simulink model "untitled"  (R2023b)
settings: Solver=VariableStepAuto  StartTime=0.0  StopTime=500  RelTol=1e-9
values from neighbouring files (symbols this model uses):
  w0 = [w0; sol]    [vetroturbina.m]
settings Model: Creator=Anja  LastModifiedBy=Anja

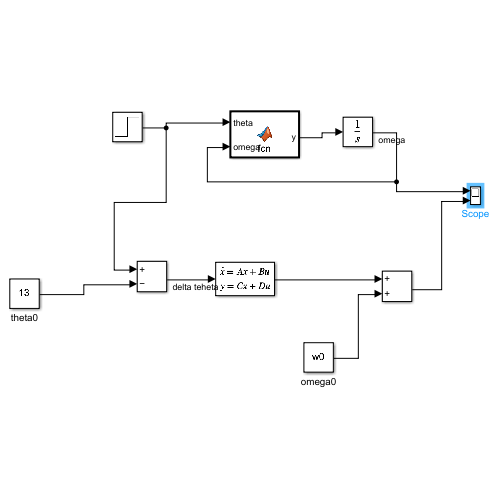
[thumbnail: Simulink's stored preview of the top-level diagram]
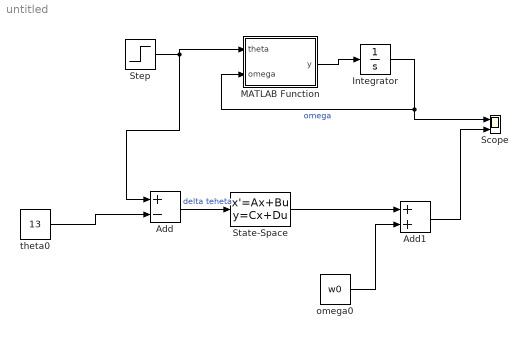
== system untitled ==
  Add : Sum  Inputs=+-
  Add1 : Sum
  Integrator : Integrator  InitialCondition=w0
  MATLAB Function : MATLAB Function  TreatAsAtomicUnit=on
  Scope : Scope  NumInputPorts=2
  State-Space : StateSpace  A=-0.1510  B=-1.4550e-05  D=0  InitialCondition=0  ParameterTunability=Unconstrained
  Step : Step  Time=0  Before=13  After=13.5  SampleTime=0
  omega0 : Constant  Value=w0
  theta0 : Constant  Value=13
  wires:
  MATLAB Function/1(y) -> Integrator/1
  theta0/1 -> Add/2
  State-Space/1 -> Add1/1
  omega0/1 -> Add1/2
  Add/1 -> State-Space/1  "delta teheta"
  Step/1 -> Add/1, MATLAB Function/1(theta)
  Integrator/1 -> Scope/1, MATLAB Function/2(omega)  "omega"
  Add1/1 -> Scope/2

== matlab function untitled/MATLAB Function ==
  data: theta input; y output; omega input
function y = fcn(theta, omega)

C1 = 0.5; 
C2 = 116; 
C3 = 0.4;
C5 = 5;
C6 = 23;
K = 160661.6;
J = 3410432;
ro = 1.225;
R = 40;
A = R*R*pi;

v = 13;
lambda = (R*omega)/v;
lambda_i = 1/(1/(lambda + 0.08*theta) - 0.035/(1 + theta^3)); 
Cp= C1*(C2/lambda_i - C3*theta - 0 - C5)*exp(-(C6/lambda_i));
   
y =(1/J)*((0.5*ro*A*Cp*(v^3))/omega - (omega^2)*K);
